simulink model "Feedback_Linearization_Controller"  (R2016a)
settings: Solver=VariableStepAuto  StartTime=0.0  StopTime=30  RelTol=1e-3
settings Model: Creator=Administrator  LastModifiedBy=Administrator

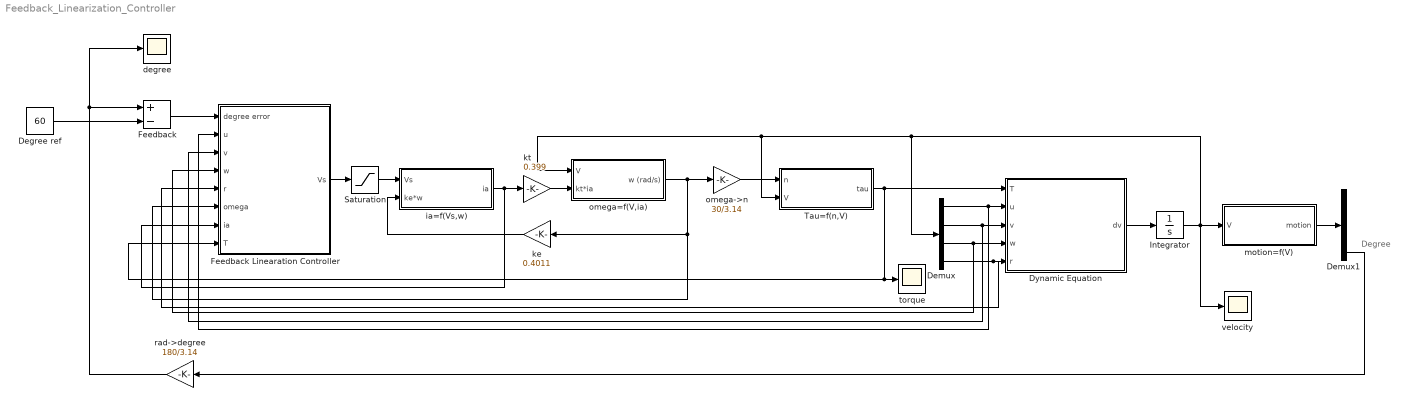
== system Feedback_Linearization_Controller ==
  note: Degree
  Degree ref : Constant  Value=60
  Demux : Demux
  Demux1 : Demux
  Dynamic Equation : MATLAB Function  TreatAsAtomicUnit=on
  Feedback : Sum  Inputs=+-
  Feedback Linearation Controller : Subsystem
  Integrator : Integrator
  Saturation : Saturate  UpperLimit=100  LowerLimit=-100
  Tau=f(n,V) : Subsystem
  degree : Scope
  ia=f(Vs,w) : Subsystem
  ke : Gain  Gain=0.4011
  kt : Gain  Gain=0.399
  motion=f(V) : Subsystem
  omega->n : Gain  Gain=30/3.14
  omega=f(V,ia) : Subsystem
  rad->degree : Gain  Gain=180/3.14
  torque : Scope
  velocity : Scope
  wires:
  ia=f(Vs,w)/1(ia) -> kt/1, Feedback Linearation Controller/7(ia)
  kt/1 -> omega=f(V,ia)/2(kt*ia)
  omega=f(V,ia)/1(w (rad/s)) -> omega->n/1, ke/1, Feedback Linearation Controller/6(omega)
  ke/1 -> ia=f(Vs,w)/2(ke*w)
  omega->n/1 -> Tau=f(n,V)/1(n)
  Tau=f(n,V)/1(tau) -> torque/1, Feedback Linearation Controller/8(T), Dynamic Equation/1(T)
  Dynamic Equation/1(dv) -> Integrator/1
  Integrator/1 -> motion=f(V)/1(V), velocity/1, Demux/1, Tau=f(n,V)/2(V), omega=f(V,ia)/1(V)
  Demux/1 -> Feedback Linearation Controller/2(u), Dynamic Equation/2(u)
  Demux/2 -> Feedback Linearation Controller/3(v), Dynamic Equation/3(v)
  Demux/3 -> Feedback Linearation Controller/4(w), Dynamic Equation/4(w)
  Demux/4 -> Feedback Linearation Controller/5(r), Dynamic Equation/5(r)
  Degree ref/1 -> Feedback/2
  motion=f(V)/1(motion) -> Demux1/1
  Demux1/4 -> rad->degree/1
  Feedback/1 -> Feedback Linearation Controller/1(degree error)
  Feedback Linearation Controller/1(Vs) -> Saturation/1
  Saturation/1 -> ia=f(Vs,w)/1(Vs)
  rad->degree/1 -> degree/1, Feedback/1

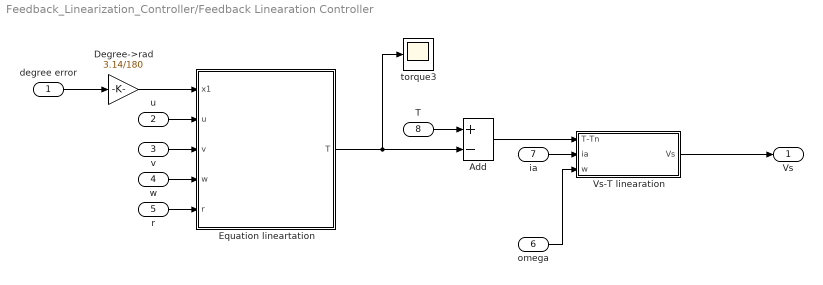
== system Feedback_Linearization_Controller/Feedback Linearation Controller ==
  degree error : Inport
  u : Inport  Port=2
  v : Inport  Port=3
  w : Inport  Port=4
  r : Inport  Port=5
  omega : Inport  Port=6
  ia : Inport  Port=7
  T : Inport  Port=8
  Add : Sum  Inputs=+-
  Degree->rad : Gain  Gain=3.14/180
  Equation lineartation : MATLAB Function  TreatAsAtomicUnit=on
  Vs-T linearation : Subsystem
  torque3 : Scope
  Vs : Outport
  wires:
  Vs-T linearation/1(Vs) -> Vs/1
  Add/1 -> Vs-T linearation/1(T-Tn)
  Equation lineartation/1(T) -> torque3/1, Add/2
  ia/1 -> Vs-T linearation/2(ia)
  omega/1 -> Vs-T linearation/3(w)
  T/1 -> Add/1
  u/1 -> Equation lineartation/2(u)
  r/1 -> Equation lineartation/5(r)
  w/1 -> Equation lineartation/4(w)
  v/1 -> Equation lineartation/3(v)
  degree error/1 -> Degree->rad/1
  Degree->rad/1 -> Equation lineartation/1(x1)

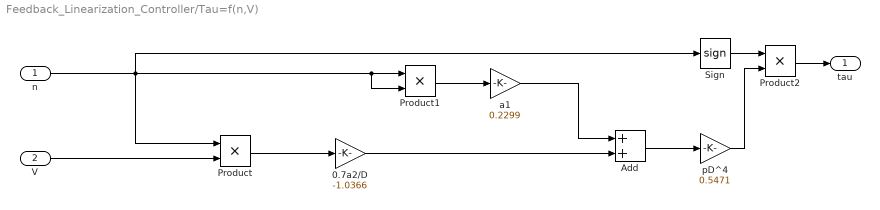
== system Feedback_Linearization_Controller/Tau=f(n,V) ==
  n : Inport
  V : Inport  Port=2
  0.7a2/D : Gain  Gain=-1.0366
  Add : Sum
  Product : Product
  Product1 : Product
  Product2 : Product
  Sign : Signum
  a1 : Gain  Gain=0.2299
  pD^4 : Gain  Gain=0.5471
  tau : Outport
  wires:
  n/1 -> Sign/1, Product/1, Product1/2, Product1/1
  V/1 -> Product/2
  Product1/1 -> a1/1
  Product/1 -> 0.7a2/D/1
  a1/1 -> Add/1
  0.7a2/D/1 -> Add/2
  Add/1 -> pD^4/1
  Sign/1 -> Product2/1
  pD^4/1 -> Product2/2
  Product2/1 -> tau/1

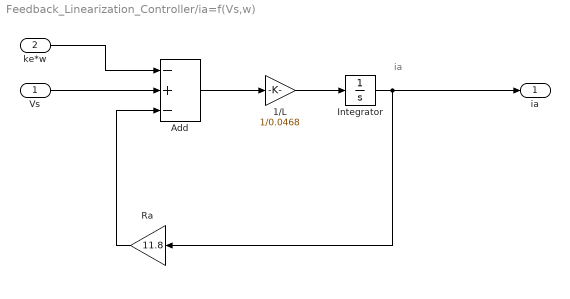
== system Feedback_Linearization_Controller/ia=f(Vs,w) ==
  note: ia
  Vs : Inport
  ke*w : Inport  Port=2
  1/L : Gain  Gain=1/0.0468
  Add : Sum  Inputs=-+-
  Integrator : Integrator
  Ra : Gain  Gain=11.8
  ia : Outport
  wires:
  Add/1 -> 1/L/1
  1/L/1 -> Integrator/1
  Integrator/1 -> ia/1, Ra/1
  Ra/1 -> Add/3
  Vs/1 -> Add/2
  ke*w/1 -> Add/1

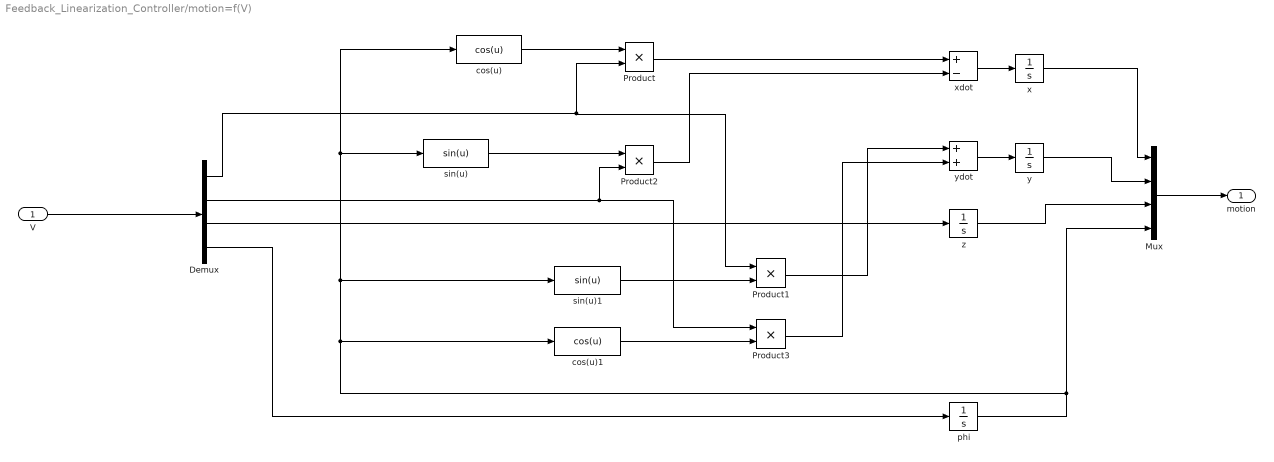
== system Feedback_Linearization_Controller/motion=f(V) ==
  V : Inport
  Demux : Demux
  Mux : Mux
  Product{,1..3} (4 alike) : Product
  cos(u) : MATLABFcn  MATLABFcn=cos(u)
  cos(u)1 : MATLABFcn  MATLABFcn=cos(u)
  phi : Integrator
  sin(u) : MATLABFcn  MATLABFcn=sin(u)
  sin(u)1 : MATLABFcn  MATLABFcn=sin(u)
  x : Integrator
  xdot : Sum  Inputs=+-
  y : Integrator
  ydot : Sum
  z : Integrator
  motion : Outport
  wires:
  V/1 -> Demux/1
  cos(u)/1 -> Product/1
  Demux/1 -> Product/2, Product1/1
  Product/1 -> xdot/1
  sin(u)/1 -> Product2/1
  Demux/2 -> Product3/1, Product2/2
  Product2/1 -> xdot/2
  sin(u)1/1 -> Product1/2
  cos(u)1/1 -> Product3/2
  Product1/1 -> ydot/1
  Product3/1 -> ydot/2
  Demux/3 -> z/1
  Demux/4 -> phi/1
  z/1 -> Mux/3
  Mux/1 -> motion/1
  phi/1 -> Mux/4, cos(u)1/1, sin(u)1/1, cos(u)/1, sin(u)/1
  xdot/1 -> x/1
  x/1 -> Mux/1
  ydot/1 -> y/1
  y/1 -> Mux/2

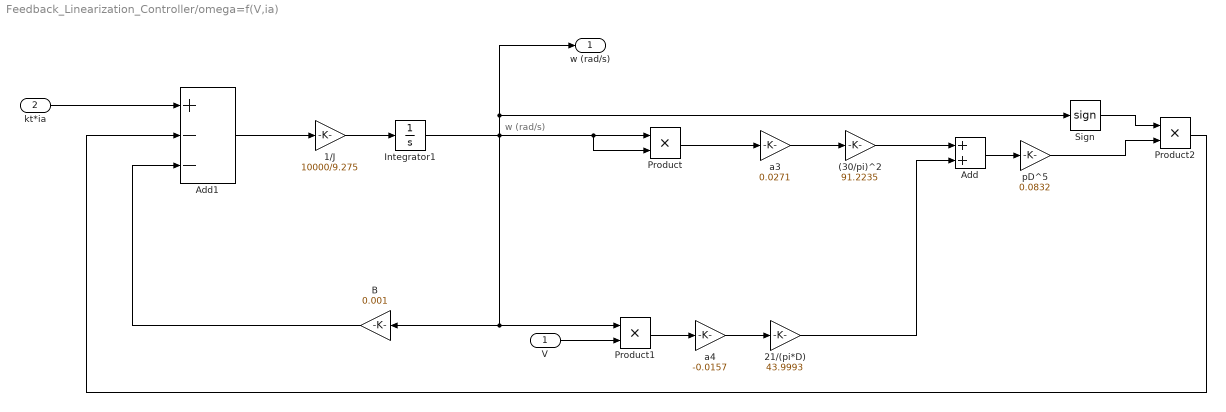
== system Feedback_Linearization_Controller/omega=f(V,ia) ==
  note: w (rad/s)
  V : Inport
  kt*ia : Inport  Port=2
  (30/pi)^2 : Gain  Gain=91.2235
  1/J : Gain  Gain=10000/9.275
  21/(pi*D) : Gain  Gain=43.9993
  Add : Sum
  Add1 : Sum  Inputs=+--
  B : Gain  Gain=0.001
  Integrator1 : Integrator
  Product : Product
  Product1 : Product
  Product2 : Product
  Sign : Signum
  a3 : Gain  Gain=0.0271
  a4 : Gain  Gain=-0.0157
  pD^5 : Gain  Gain=0.0832
  w (rad/s) : Outport
  wires:
  1/J/1 -> Integrator1/1
  Add1/1 -> 1/J/1
  B/1 -> Add1/3
  Integrator1/1 -> Product/2, Product/1, w (rad/s)/1, Sign/1, Product1/1, B/1
  kt*ia/1 -> Add1/1
  Product/1 -> a3/1
  a3/1 -> (30/pi)^2/1
  (30/pi)^2/1 -> Add/1
  a4/1 -> 21/(pi*D)/1
  V/1 -> Product1/2
  Product1/1 -> a4/1
  21/(pi*D)/1 -> Add/2
  Add/1 -> pD^5/1
  Sign/1 -> Product2/1
  pD^5/1 -> Product2/2
  Product2/1 -> Add1/2

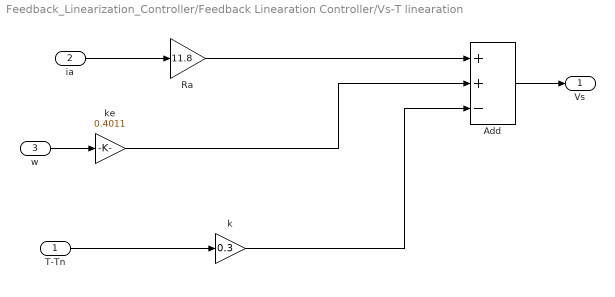
== system Feedback_Linearization_Controller/Feedback Linearation Controller/Vs-T linearation ==
  T-Tn : Inport
  ia : Inport  Port=2
  w : Inport  Port=3
  Add : Sum  Inputs=++-
  Ra : Gain  Gain=11.8
  k : Gain  Gain=0.3
  ke : Gain  Gain=0.4011
  Vs : Outport
  wires:
  ia/1 -> Ra/1
  Ra/1 -> Add/1
  w/1 -> ke/1
  ke/1 -> Add/2
  Add/1 -> Vs/1
  T-Tn/1 -> k/1
  k/1 -> Add/3

== matlab function Feedback_Linearization_Controller/Dynamic Equation ==
  data: T input; dv output; u input; v input; w input; r input
function dv = fcn(T,u,v,w,r)
%#codegen

%%velocity
vel=[u;v;w;r];
%% propeller
D=0.152;

%% motor
J=9.275*1e-4;
ke=0.4011;
Ra=11.8;
L=0.0468;
kt=0.399;
B=0.001;
m=128;
g=9.8;

%%cordinate
xG=0;yG=0;zG=0.054;
Iz=14.213;

%%matirx
Mrb=[m 0 0 -m*yG;0 m 0 m*xG;0 0 m 0;-m*yG m*xG 0 Iz];
Ma=-1*[-33.48 0 0 0;0 -110.8941 0 -4.921;0 0 -147.576 0;0 -4.921 0 -12.75];
Crb=-1*[0 0 0 -m*(xG*r+v);0 0 0 -m*(yG*r-u);0 0 0 0;m*(xG*r+v) m*(yG*r-u) 0 0];
Ca=-1*[0 0 0 -110.8941*v-4.921*r;0 0 0 33.48*u;0 0 0 0;110.8941*v+4.921*r -33.48*u 0 0];
Dv=-1*[-4.9217-139.8007*abs(u) 0 0 0;0 -3.0591-350.2618*abs(v) 0 0;0 0 -4.4132-327.2375*abs(w) 0;0 0 0 -1.3881-51.1709*abs(r)];
G=[0;0;0;0];

%% Equation
tau=T;

dvel=(Mrb+Ma)^(-1)*(tau-G-(Crb+Ca+Dv)*vel);  %% state equation

%%output
dv=dvel;

== matlab function Feedback_Linearization_Controller/Feedback Linearation Controller/Equation lineartation ==
  data: x1 input; u input; v input; w input; T output; r input
function T = fcn(x1,u,v,w,r)
%#codegen

%%velocity
vel=[u;v;w;r];
%% propeller
D=0.152;

%% motor
J=9.275*1e-4;
ke=0.4011;
Ra=11.8;
L=0.0468;
kt=0.399;
B=0.001;
m=128;
g=9.8;

%%cordinate
xG=0;yG=0;zG=0.054;
Iz=14.213;

%%matirx
Mrb=[m 0 0 -m*yG;0 m 0 m*xG;0 0 m 0;-m*yG m*xG 0 Iz];
Ma=-1*[-33.48 0 0 0;0 -110.8941 0 -4.921;0 0 -147.576 0;0 -4.921 0 -12.75];
Crb=-1*[0 0 0 -m*(xG*r+v);0 0 0 -m*(yG*r-u);0 0 0 0;m*(xG*r+v) m*(yG*r-u) 0 0];
Ca=-1*[0 0 0 -110.8941*v-4.921*r;0 0 0 33.48*u;0 0 0 0;110.8941*v+4.921*r -33.48*u 0 0];
Dv=-1*[-4.9217-139.8007*abs(u) 0 0 0;0 -3.0591-350.2618*abs(v) 0 0;0 0 -4.4132-327.2375*abs(w) 0;0 0 0 -1.3881-51.1709*abs(r)];
G=[0;0;0;0];


%% Lineartion
N=Crb+Ca+Dv;
A=Mrb+Ma;

Mz=A*[u;v;w;-0.3*x1-1*r];
a=N*vel;

a(4)+Mz(4); %%Choose Mz as U,then linearize

%%output
T=[0;0;0;a(4)+Mz(4)];
